simulink model "viewer_simulink"  (R2023a)
settings: Solver=VariableStepAuto  StartTime=0.0  StopTime=inf  RelTol=1e-3
undefined symbols (not defined in the file or in its folder): hl2ss
libraries: matrix_library x14, visionsinks x9, visionanalysis x4
settings Model: Creator=jcds  LastModifiedBy=jcds

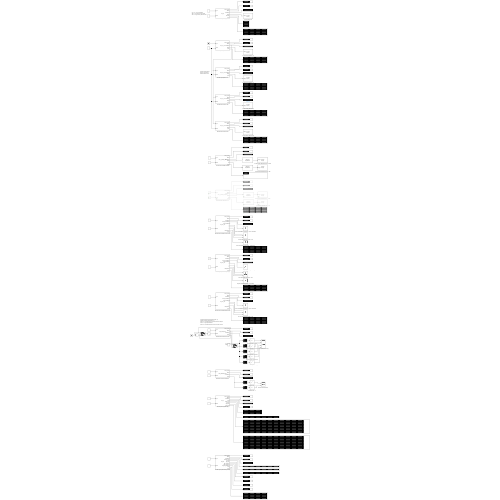
[thumbnail: Simulink's stored preview of the top-level diagram]
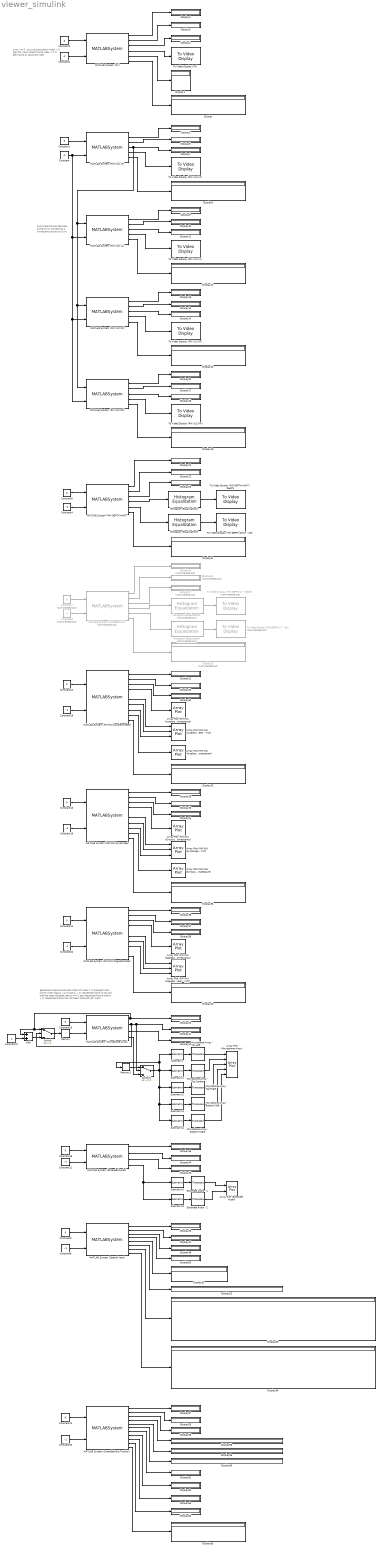
== system viewer_simulink ==
  note: Sequential capture example (start at index = 0)
      | Request next frame when status <= 0
      | status < 0: requested frame is too old and has been dropped
      | status == 0: got requested frame
      | status < 0: requested frame has not been received yet (wait)
  note: Associate frames between streams by connecting a timestamp output to sync
  note: sync <= 0 : no synchronization
      | index < 0: get nth most recent frame
      | index >= 0: get frame by absolute index
  Add : Sum
  Array Plot (Extended Audio) : ArrayPlot  NumInputPorts=2  WindowPosition=[158.000000,113.000000,800.000000,500.000000,]  Visible=on  ScopeFrameLocation=window  YLimits=[-0.0094,0.0077]  ShowLegend=on
  Array Plot (Microphone Array) : ArrayPlot  NumInputPorts=5  WindowPosition=[1013.000000,246.000000,800.000000,500.000000,]  Visible=on  ScopeFrameLocation=window  YLimits=[-0.0014,0.002]  ShowLegend=on
  Array Plot (RM IMU Accelerometer - Temperature) : ArrayPlot  WindowPosition=[770.000000,171.000000,800.000000,456.000000,]  Visible=on  ScopeFrameLocation=window  YLimits=[42.1563,54.2813]
  Array Plot (RM IMU Accelerometer - XYZ) : ArrayPlot  NumInputPorts=3  WindowPosition=[710.000000,401.000000,800.000000,500.000000,]  Visible=on  ScopeFrameLocation=window  YLimits=[-2.1398,11.1348]  ShowLegend=on
  Array Plot (RM IMU Accelerometer - sensor_timestamp) : ArrayPlot  WindowPosition=[1090.000000,48.000000,800.000000,456.000000,]  Visible=on  ScopeFrameLocation=window  YLimits=[302887973136.125,302992202644.875]
  Array Plot (RM IMU Gyroscope - Temperature) : ArrayPlot  WindowPosition=[770.000000,171.000000,800.000000,456.000000,]  Visible=on  ScopeFrameLocation=window  YLimits=[37.4858,48.2212]
  Array Plot (RM IMU Gyroscope - XYZ) : ArrayPlot  NumInputPorts=3  WindowPosition=[692.000000,115.000000,800.000000,500.000000,]  Visible=on  ScopeFrameLocation=window  YLimits=[-0.1057,0.1007]  ShowLegend=on
  Array Plot (RM IMU Gyroscope - sensor_timestamp) : ArrayPlot  WindowPosition=[1090.000000,48.000000,800.000000,456.000000,]  Visible=on  ScopeFrameLocation=window  YLimits=[302821386482.875,302881349464.125]
  Array Plot (RM IMU Magnetometer - XYZ) : ArrayPlot  NumInputPorts=3  WindowPosition=[952.000000,106.000000,800.000000,500.000000,]  Visible=on  ScopeFrameLocation=window  YLimits=[-377.475,569.775]  ShowLegend=on
  Array Plot (RM IMU Magnetometer - sensor_timestamp) : ArrayPlot  WindowPosition=[983.000000,49.000000,800.000000,456.000000,]  Visible=on  ScopeFrameLocation=window  YLimits=[302697878061.125,302947875559.875]
  Constant{,2,4,8,10,18..21} (9 alike) : Constant  Value=-1
  Constant{1,3,5,9,11..16} (10 alike) : Constant  Value=0
  Constant17 : Constant  OutDataTypeStr=int64
  Constant6 : Constant  Commented=on  Value=-1
  Constant7 : Constant  Commented=on  Value=0
  Display{,1..24,29..65} (62 alike) : Display
  Display{25..28} (4 alike) : Display  Commented=on
  Extended Audio - 1 : matrix_library/Transpose
  Extended Audio - 2 : matrix_library/Transpose
  Histogram Equalization : visionanalysis/Histogram Equalization  Commented=on  specify=Uniform  numbins=64  src=Specify via dialog  hist=ones(1,64)
  Histogram Equalization1 : visionanalysis/Histogram Equalization  Commented=on  specify=Uniform  numbins=64  src=Specify via dialog  hist=ones(1,64)
  Histogram Equalization2 : visionanalysis/Histogram Equalization  specify=Uniform  numbins=64  src=Specify via dialog  hist=ones(1,64)
  Histogram Equalization3 : visionanalysis/Histogram Equalization  specify=Uniform  numbins=64  src=Specify via dialog  hist=ones(1,64)
  MATLAB System (Extended Audio) : MATLABSystem  System=hl2ss.ms.sink_extended_audio  host=192.168.1.7  port=hl2ss.stream_port.EXTENDED_AUDIO  chunk=4096  mixer_mode=hl2ss.mixer_mode.BOTH  device=-1  loopback_gain=1.0  microphone_gain=1.0  profile=hl2ss.audio_profile.AAC_24000  level=hl2ss.aac_level.L2  buffer_size=1000  sample_time=hl2ss.parameters_microphone.GROUP_SIZE_AAC / hl2ss.parameters_microphone.SAMPLE_RATE  time_preference=hl2ss.grab_preference.PREFER_NEAREST  tiebreak_right=false  SimulateUsing=Code generation
      mask Type: hl2ss.ms.sink_extended_audio
      mask Display:
      | disp('sink_extended_audio');
      | port_label('input',1,'sync');
      | port_label('input',2,'index');
      | port_label('output',1,'frame_index');
      | port_label('output',2,'status');
      | port_label('output',3,'timestamp');
      | port_label('output',4,'audio');
  MATLAB System (Extended Eye Tracker) : MATLABSystem  System=hl2ss.ms.sink_eet  host=192.168.1.7  port=hl2ss.stream_port.EXTENDED_EYE_TRACKER  chunk=4096  framerate=90  buffer_size=300  sample_time=1 / 90  time_preference=hl2ss.grab_preference.PREFER_NEAREST  tiebreak_right=false  SimulateUsing=Code generation
      mask Type: hl2ss.ms.sink_eet
      mask Display:
      | disp('sink_eet');
      | port_label('input',1,'sync');
      | port_label('input',2,'index');
      | port_label('output',1,'frame_index');
      | port_label('output',2,'status');
      | port_label('output',3,'timestamp');
      | port_label('output',4,'combined_ray');
      | port_label('output',5,'left_ray');
      | port_label('output',6,'right_ray');
      | port_label('output',7,'left_openness');
      | port_label('output',8,'right_openness');
      | port_label('output',9,'vergence_distance');
      | port_label('output',10,'valid');
      | port_label('output',11,'pose');
  MATLAB System (Microphone Array) : MATLABSystem  System=hl2ss.ms.sink_microphone  host=192.168.1.7  port=hl2ss.stream_port.MICROPHONE  chunk=4096  profile=hl2ss.audio_profile.RAW  level=hl2ss.aac_level.L5  buffer_size=1000  sample_time=hl2ss.parameters_microphone.GROUP_SIZE_RAW / hl2ss.parameters_microphone.SAMPLE_RATE  time_preference=hl2ss.grab_preference.PREFER_NEAREST  tiebreak_right=false  SimulateUsing=Code generation
      mask Type: hl2ss.ms.sink_microphone
      mask Display:
      | disp('sink_microphone');
      | port_label('input',1,'sync');
      | port_label('input',2,'index');
      | port_label('output',1,'frame_index');
      | port_label('output',2,'status');
      | port_label('output',3,'timestamp');
      | port_label('output',4,'audio');
  MATLAB System (PV) : MATLABSystem  System=hl2ss.ms.sink_pv  host=192.168.1.7  port=hl2ss.stream_port.PERSONAL_VIDEO  width=640  height=360  framerate=30  chunk=4096  mode=hl2ss.stream_mode.MODE_1  divisor=1  profile=hl2ss.video_profile.H265_MAIN  level=hl2ss.h26x_level.DEFAULT  bitrate=0  options=[ hl2ss.h26x_encoder_property.CODECAPI_AVEncMPVGOPSize, 30 ]  decoded_format=hl2ss.pv_decoded_format.RGB  buffer_size=30 * 10  sample_time=1 / 30  enable_mrc=false  hologram_composition=true  recording_indicator=false  video_stabilization=false  blank_protected=false  show_mesh=false  shared=false  global_opacity=0.9  output_width=0.0  output_height=0.0  video_stabilization_length=0  hologram_perspective=hl2ss.hologram_perspective.PV  time_preference=hl2ss.grab_preference.PREFER_NEAREST  tiebreak_right=false  SimulateUsing=Code generation
      mask Type: hl2ss.ms.sink_pv
      mask Display:
      | disp('sink_pv');
      | port_label('input',1,'sync');
      | port_label('input',2,'index');
      | port_label('output',1,'frame_index');
      | port_label('output',2,'status');
      | port_label('output',3,'timestamp');
      | port_label('output',4,'image');
      | port_label('output',5,'intrinsics');
      | port_label('output',6,'pose');
  MATLAB System (RM DEPTH AHAT) : MATLABSystem  System=hl2ss.ms.sink_rm_depth_ahat  host=192.168.1.7  port=hl2ss.stream_port.RM_DEPTH_AHAT  chunk=4096  mode=hl2ss.stream_mode.MODE_1  divisor=1  profile_z=hl2ss.depth_profile.SAME  profile_ab=hl2ss.video_profile.H265_MAIN  level=hl2ss.h26x_level.DEFAULT  bitrate=0  options=[ hl2ss.h26x_encoder_property.CODECAPI_AVEncMPVGOPSize, hl2ss.parameters_rm_depth_ahat.FPS ]  buffer_size=hl2ss.parameters_rm_depth_ahat.FPS * 10  sample_time=1 / hl2ss.parameters_rm_depth_ahat.FPS  time_preference=hl2ss.grab_preference.PREFER_NEAREST  tiebreak_right=false  SimulateUsing=Code generation
      mask Type: hl2ss.ms.sink_rm_depth_ahat
      mask Display:
      | disp('sink_rm_depth_ahat');
      | port_label('input',1,'sync');
      | port_label('input',2,'index');
      | port_label('output',1,'frame_index');
      | port_label('output',2,'status');
      | port_label('output',3,'timestamp');
      | port_label('output',4,'depth');
      | port_label('output',5,'ab');
      | port_label('output',6,'pose');
  MATLAB System (RM DEPTH LT) : MATLABSystem  Commented=on  System=hl2ss.ms.sink_rm_depth_longthrow  host=192.168.1.7  port=hl2ss.stream_port.RM_DEPTH_LONGTHROW  chunk=4096  mode=hl2ss.stream_mode.MODE_1  divisor=1  png_filter=hl2ss.png_filter_mode.PAETH  buffer_size=hl2ss.parameters_rm_depth_longthrow.FPS * 10  sample_time=1 / hl2ss.parameters_rm_depth_longthrow.FPS  time_preference=hl2ss.grab_preference.PREFER_NEAREST  tiebreak_right=false  SimulateUsing=Code generation
      mask Type: hl2ss.ms.sink_rm_depth_longthrow
      mask Display:
      | disp('sink_rm_depth_longthrow');
      | port_label('input',1,'sync');
      | port_label('input',2,'index');
      | port_label('output',1,'frame_index');
      | port_label('output',2,'status');
      | port_label('output',3,'timestamp');
      | port_label('output',4,'depth');
      | port_label('output',5,'ab');
      | port_label('output',6,'pose');
  MATLAB System (RM IMU Accelerometer) : MATLABSystem  System=hl2ss.ms.sink_rm_imu  host=192.168.1.7  port=hl2ss.stream_port.RM_IMU_ACCELEROMETER  chunk=4096  mode=hl2ss.stream_mode.MODE_1  buffer_size=300  sample_time=1 / 30  time_preference=hl2ss.grab_preference.PREFER_NEAREST  tiebreak_right=false  SimulateUsing=Code generation
      mask Type: hl2ss.ms.sink_rm_imu
      mask Display:
      | disp('sink_rm_imu');
      | port_label('input',1,'sync');
      | port_label('input',2,'index');
      | port_label('output',1,'frame_index');
      | port_label('output',2,'status');
      | port_label('output',3,'timestamp');
      | port_label('output',4,'sensor_timestamp');
      | port_label('output',5,'host_timestamp');
      | port_label('output',6,'x');
      | port_label('output',7,'y');
      | port_label('output',8,'z');
      | port_label('output',9,'temperature');
      | port_label('output',10,'pose');
  MATLAB System (RM IMU Gyroscope) : MATLABSystem  System=hl2ss.ms.sink_rm_imu  host=192.168.1.7  port=hl2ss.stream_port.RM_IMU_GYROSCOPE  chunk=4096  mode=hl2ss.stream_mode.MODE_1  buffer_size=300  sample_time=1 / 30  time_preference=hl2ss.grab_preference.PREFER_NEAREST  tiebreak_right=false  SimulateUsing=Code generation
      mask Type: hl2ss.ms.sink_rm_imu
      mask Display:
      | disp('sink_rm_imu');
      | port_label('input',1,'sync');
      | port_label('input',2,'index');
      | port_label('output',1,'frame_index');
      | port_label('output',2,'status');
      | port_label('output',3,'timestamp');
      | port_label('output',4,'sensor_timestamp');
      | port_label('output',5,'host_timestamp');
      | port_label('output',6,'x');
      | port_label('output',7,'y');
      | port_label('output',8,'z');
      | port_label('output',9,'temperature');
      | port_label('output',10,'pose');
  MATLAB System (RM IMU Magnetometer) : MATLABSystem  System=hl2ss.ms.sink_rm_imu  host=192.168.1.7  port=hl2ss.stream_port.RM_IMU_MAGNETOMETER  chunk=4096  mode=hl2ss.stream_mode.MODE_1  buffer_size=300  sample_time=1 / 30  time_preference=hl2ss.grab_preference.PREFER_NEAREST  tiebreak_right=false  SimulateUsing=Code generation
      mask Type: hl2ss.ms.sink_rm_imu
      mask Display:
      | disp('sink_rm_imu');
      | port_label('input',1,'sync');
      | port_label('input',2,'index');
      | port_label('output',1,'frame_index');
      | port_label('output',2,'status');
      | port_label('output',3,'timestamp');
      | port_label('output',4,'sensor_timestamp');
      | port_label('output',5,'host_timestamp');
      | port_label('output',6,'x');
      | port_label('output',7,'y');
      | port_label('output',8,'z');
      | port_label('output',9,'temperature');
      | port_label('output',10,'pose');
  MATLAB System (RM VLC LF) : MATLABSystem  System=hl2ss.ms.sink_rm_vlc  host=192.168.1.7  port=hl2ss.stream_port.RM_VLC_LEFTFRONT  chunk=4096  mode=hl2ss.stream_mode.MODE_1  divisor=1  profile=hl2ss.video_profile.H265_MAIN  level=hl2ss.h26x_level.DEFAULT  bitrate=0  options=[ hl2ss.h26x_encoder_property.CODECAPI_AVEncMPVGOPSize, 30 ]  buffer_size=300  sample_time=1 / 30  time_preference=hl2ss.grab_preference.PREFER_NEAREST  tiebreak_right=false  SimulateUsing=Code generation
      mask Type: hl2ss.ms.sink_rm_vlc
      mask Display:
      | disp('sink_rm_vlc');
      | port_label('input',1,'sync');
      | port_label('input',2,'index');
      | port_label('output',1,'frame_index');
      | port_label('output',2,'status');
      | port_label('output',3,'timestamp');
      | port_label('output',4,'image');
      | port_label('output',5,'pose');
  MATLAB System (RM VLC LL) : MATLABSystem  System=hl2ss.ms.sink_rm_vlc  host=192.168.1.7  port=hl2ss.stream_port.RM_VLC_LEFTLEFT  chunk=4096  mode=hl2ss.stream_mode.MODE_1  divisor=1  profile=hl2ss.video_profile.H265_MAIN  level=hl2ss.h26x_level.DEFAULT  bitrate=0  options=[ hl2ss.h26x_encoder_property.CODECAPI_AVEncMPVGOPSize, 30 ]  buffer_size=300  sample_time=1 / 30  time_preference=hl2ss.grab_preference.PREFER_NEAREST  tiebreak_right=false  SimulateUsing=Code generation
      mask Type: hl2ss.ms.sink_rm_vlc
      mask Display:
      | disp('sink_rm_vlc');
      | port_label('input',1,'sync');
      | port_label('input',2,'index');
      | port_label('output',1,'frame_index');
      | port_label('output',2,'status');
      | port_label('output',3,'timestamp');
      | port_label('output',4,'image');
      | port_label('output',5,'pose');
  MATLAB System (RM VLC RF) : MATLABSystem  System=hl2ss.ms.sink_rm_vlc  host=192.168.1.7  port=hl2ss.stream_port.RM_VLC_RIGHTFRONT  chunk=4096  mode=hl2ss.stream_mode.MODE_1  divisor=1  profile=hl2ss.video_profile.H265_MAIN  level=hl2ss.h26x_level.DEFAULT  bitrate=0  options=[ hl2ss.h26x_encoder_property.CODECAPI_AVEncMPVGOPSize, 30 ]  buffer_size=300  sample_time=1 / 30  time_preference=hl2ss.grab_preference.PREFER_NEAREST  tiebreak_right=false  SimulateUsing=Code generation
      mask Type: hl2ss.ms.sink_rm_vlc
      mask Display:
      | disp('sink_rm_vlc');
      | port_label('input',1,'sync');
      | port_label('input',2,'index');
      | port_label('output',1,'frame_index');
      | port_label('output',2,'status');
      | port_label('output',3,'timestamp');
      | port_label('output',4,'image');
      | port_label('output',5,'pose');
  MATLAB System (RM VLC RR) : MATLABSystem  System=hl2ss.ms.sink_rm_vlc  host=192.168.1.7  port=hl2ss.stream_port.RM_VLC_RIGHTRIGHT  chunk=4096  mode=hl2ss.stream_mode.MODE_1  divisor=1  profile=hl2ss.video_profile.H265_MAIN  level=hl2ss.h26x_level.DEFAULT  bitrate=0  options=[ hl2ss.h26x_encoder_property.CODECAPI_AVEncMPVGOPSize, 30 ]  buffer_size=300  sample_time=1 / 30  time_preference=hl2ss.grab_preference.PREFER_NEAREST  tiebreak_right=false  SimulateUsing=Code generation
      mask Type: hl2ss.ms.sink_rm_vlc
      mask Display:
      | disp('sink_rm_vlc');
      | port_label('input',1,'sync');
      | port_label('input',2,'index');
      | port_label('output',1,'frame_index');
      | port_label('output',2,'status');
      | port_label('output',3,'timestamp');
      | port_label('output',4,'image');
      | port_label('output',5,'pose');
  MATLAB System (Spatial Input) : MATLABSystem  System=hl2ss.ms.sink_si  host=192.168.1.7  port=hl2ss.stream_port.SPATIAL_INPUT  chunk=4096  buffer_size=300  sample_time=1 / hl2ss.parameters_si.SAMPLE_RATE  time_preference=hl2ss.grab_preference.PREFER_NEAREST  tiebreak_right=false  SimulateUsing=Code generation
      mask Type: hl2ss.ms.sink_si
      mask Display:
      | disp('sink_si');
      | port_label('input',1,'sync');
      | port_label('input',2,'index');
      | port_label('output',1,'frame_index');
      | port_label('output',2,'status');
      | port_label('output',3,'timestamp');
      | port_label('output',4,'valid');
      | port_label('output',5,'head_pose');
      | port_label('output',6,'eye_ray');
      | port_label('output',7,'left_hand');
      | port_label('output',8,'right_hand');
  Memory : Memory
  Memory1 : Memory
  Microphone Array - Bottom Left : matrix_library/Transpose
  Microphone Array - Bottom Right : matrix_library/Transpose
  Microphone Array - Top Center : matrix_library/Transpose
  Microphone Array - Top Left : matrix_library/Transpose
  Microphone Array - Top Right : matrix_library/Transpose
  Submatrix : matrix_library/Submatrix  RowSpan=One row  RowStartMode=Index  RowStartIndex=1  RowEndMode=Last  RowEndIndex=1  ColSpan=All columns  ColStartMode=First  ColStartIndex=1  ColEndMode=Last  ColEndIndex=1
  Submatrix1 : matrix_library/Submatrix  RowSpan=One row  RowStartMode=Index  RowStartIndex=2  RowEndMode=Last  RowEndIndex=1  ColSpan=All columns  ColStartMode=First  ColStartIndex=1  ColEndMode=Last  ColEndIndex=1
  Submatrix2 : matrix_library/Submatrix  RowSpan=One row  RowStartMode=Index  RowStartIndex=3  RowEndMode=Last  RowEndIndex=1  ColSpan=All columns  ColStartMode=First  ColStartIndex=1  ColEndMode=Last  ColEndIndex=1
  Submatrix3 : matrix_library/Submatrix  RowSpan=One row  RowStartMode=Index  RowStartIndex=4  RowEndMode=Last  RowEndIndex=1  ColSpan=All columns  ColStartMode=First  ColStartIndex=1  ColEndMode=Last  ColEndIndex=1
  Submatrix4 : matrix_library/Submatrix  RowSpan=One row  RowStartMode=Index  RowStartIndex=5  RowEndMode=Last  RowEndIndex=1  ColSpan=All columns  ColStartMode=First  ColStartIndex=1  ColEndMode=Last  ColEndIndex=1
  Submatrix5 : matrix_library/Submatrix  RowSpan=One row  RowStartMode=Index  RowStartIndex=1  RowEndMode=Last  RowEndIndex=1  ColSpan=All columns  ColStartMode=First  ColStartIndex=1  ColEndMode=Last  ColEndIndex=1
  Submatrix6 : matrix_library/Submatrix  RowSpan=One row  RowStartMode=Index  RowStartIndex=2  RowEndMode=Last  RowEndIndex=1  ColSpan=All columns  ColStartMode=First  ColStartIndex=1  ColEndMode=Last  ColEndIndex=1
  Switch : Switch  Criteria=u2 > Threshold  SaturateOnIntegerOverflow=off  InputSameDT=off
  Switch1 : Switch  Criteria=u2 ~= 0  SaturateOnIntegerOverflow=off  InputSameDT=off
  To Video Display (PV) : visionsinks/To Video Display  windowSizeMode=Normal  openAtMdlStart=on  fullScreen=off  videoWindowX=2170  videoWindowY=212  saveWindowSize=off  videoWindowWidth=640  videoWindowHeight=360  inputColorFormat=RGB  inputType=Obsolete  imagePorts=One multidimensional signal  OutputDevice=On-screen video monitor  dataOrg=Column-major  isWindowOpen=off
  To Video Display (RM DEPTH AHAT - AB) : visionsinks/To Video Display  windowSizeMode=Normal  openAtMdlStart=on  fullScreen=off  videoWindowX=2573  videoWindowY=991  saveWindowSize=off  videoWindowWidth=744  videoWindowHeight=668  inputColorFormat=RGB  inputType=Obsolete  imagePorts=One multidimensional signal  OutputDevice=On-screen video monitor  dataOrg=Column-major  isWindowOpen=off
  To Video Display (RM DEPTH AHAT - Depth) : visionsinks/To Video Display  windowSizeMode=Normal  openAtMdlStart=on  fullScreen=off  videoWindowX=1597  videoWindowY=1025  saveWindowSize=off  videoWindowWidth=829  videoWindowHeight=727  inputColorFormat=RGB  inputType=Obsolete  imagePorts=One multidimensional signal  OutputDevice=On-screen video monitor  dataOrg=Column-major  isWindowOpen=off
  To Video Display (RM DEPTH LT - AB) : visionsinks/To Video Display  Commented=on  windowSizeMode=Normal  openAtMdlStart=on  fullScreen=off  videoWindowX=917  videoWindowY=1195  saveWindowSize=off  videoWindowWidth=512  videoWindowHeight=512  inputColorFormat=RGB  inputType=Obsolete  imagePorts=One multidimensional signal  OutputDevice=On-screen video monitor  dataOrg=Column-major  isWindowOpen=off
  To Video Display (RM DEPTH LT - Depth) : visionsinks/To Video Display  Commented=on  windowSizeMode=Normal  openAtMdlStart=on  fullScreen=off  videoWindowX=1462  videoWindowY=1164  saveWindowSize=off  videoWindowWidth=512  videoWindowHeight=512  inputColorFormat=RGB  inputType=Obsolete  imagePorts=One multidimensional signal  OutputDevice=On-screen video monitor  dataOrg=Column-major  isWindowOpen=off
  To Video Display (RM VLC LF) : visionsinks/To Video Display  windowSizeMode=Normal  openAtMdlStart=on  fullScreen=off  videoWindowX=2960  videoWindowY=641  saveWindowSize=off  videoWindowWidth=781  videoWindowHeight=480  inputColorFormat=RGB  inputType=Obsolete  imagePorts=One multidimensional signal  OutputDevice=On-screen video monitor  dataOrg=Column-major  isWindowOpen=off
  To Video Display (RM VLC LL) : visionsinks/To Video Display  windowSizeMode=Normal  openAtMdlStart=on  fullScreen=off  videoWindowX=2971  videoWindowY=101  saveWindowSize=off  videoWindowWidth=781  videoWindowHeight=480  inputColorFormat=RGB  inputType=Obsolete  imagePorts=One multidimensional signal  OutputDevice=On-screen video monitor  dataOrg=Column-major  isWindowOpen=off
  To Video Display (RM VLC RF) : visionsinks/To Video Display  windowSizeMode=Normal  openAtMdlStart=on  fullScreen=off  videoWindowX=2330  videoWindowY=1248  saveWindowSize=off  videoWindowWidth=781  videoWindowHeight=480  inputColorFormat=RGB  inputType=Obsolete  imagePorts=One multidimensional signal  OutputDevice=On-screen video monitor  dataOrg=Column-major  isWindowOpen=off
  To Video Display (RM VLC RR) : visionsinks/To Video Display  windowSizeMode=Normal  openAtMdlStart=on  fullScreen=off  videoWindowX=2962  videoWindowY=1176  saveWindowSize=off  videoWindowWidth=781  videoWindowHeight=480  inputColorFormat=RGB  inputType=Obsolete  imagePorts=One multidimensional signal  OutputDevice=On-screen video monitor  dataOrg=Column-major  isWindowOpen=off
  wires:
  MATLAB System (PV)/4 -> To Video Display (PV)/1
  MATLAB System (PV)/6 -> Display/1
  MATLAB System (PV)/5 -> Display1/1
  MATLAB System (PV)/3 -> Display2/1
  MATLAB System (PV)/2 -> Display3/1
  MATLAB System (PV)/1 -> Display4/1
  MATLAB System (RM VLC LF)/4 -> To Video Display (RM VLC LF)/1
  MATLAB System (RM VLC LF)/1 -> Display5/1
  MATLAB System (RM VLC LF)/2 -> Display6/1
  MATLAB System (RM VLC LF)/3 -> MATLAB System (RM VLC RR)/1, MATLAB System (RM VLC RF)/1, MATLAB System (RM VLC LL)/1, Display7/1
  MATLAB System (RM VLC LF)/5 -> Display8/1
  MATLAB System (RM VLC LL)/5 -> Display12/1
  MATLAB System (RM VLC LL)/3 -> Display11/1
  MATLAB System (RM VLC LL)/4 -> To Video Display (RM VLC LL)/1
  MATLAB System (RM VLC LL)/2 -> Display10/1
  MATLAB System (RM VLC LL)/1 -> Display9/1
  MATLAB System (RM VLC RF)/3 -> Display14/1
  MATLAB System (RM VLC RF)/4 -> To Video Display (RM VLC RF)/1
  MATLAB System (RM VLC RF)/1 -> Display16/1
  MATLAB System (RM VLC RF)/2 -> Display13/1
  MATLAB System (RM VLC RF)/5 -> Display15/1
  MATLAB System (RM VLC RR)/3 -> Display18/1
  MATLAB System (RM VLC RR)/1 -> Display20/1
  MATLAB System (RM VLC RR)/4 -> To Video Display (RM VLC RR)/1
  MATLAB System (RM VLC RR)/5 -> Display19/1
  MATLAB System (RM VLC RR)/2 -> Display17/1
  MATLAB System (RM DEPTH AHAT)/6 -> Display21/1
  MATLAB System (RM DEPTH AHAT)/2 -> Display22/1
  MATLAB System (RM DEPTH AHAT)/3 -> Display23/1
  MATLAB System (RM DEPTH AHAT)/1 -> Display24/1
  MATLAB System (RM DEPTH LT)/2 -> Display26/1
  MATLAB System (RM DEPTH LT)/1 -> Display28/1
  MATLAB System (RM DEPTH LT)/6 -> Display25/1
  MATLAB System (RM DEPTH LT)/3 -> Display27/1
  MATLAB System (RM DEPTH LT)/5 -> Histogram Equalization/1
  Histogram Equalization/1 -> To Video Display (RM DEPTH LT - AB)/1
  Histogram Equalization1/1 -> To Video Display (RM DEPTH LT - Depth)/1
  MATLAB System (RM DEPTH LT)/4 -> Histogram Equalization1/1
  Histogram Equalization2/1 -> To Video Display (RM DEPTH AHAT - Depth)/1
  Histogram Equalization3/1 -> To Video Display (RM DEPTH AHAT - AB)/1
  MATLAB System (RM DEPTH AHAT)/4 -> Histogram Equalization2/1
  MATLAB System (RM DEPTH AHAT)/5 -> Histogram Equalization3/1
  MATLAB System (RM IMU Accelerometer)/1 -> Display31/1
  MATLAB System (RM IMU Accelerometer)/2 -> Display29/1
  MATLAB System (RM IMU Accelerometer)/3 -> Display30/1
  MATLAB System (RM IMU Accelerometer)/6 -> Array Plot (RM IMU Accelerometer - XYZ)/1
  MATLAB System (RM IMU Accelerometer)/7 -> Array Plot (RM IMU Accelerometer - XYZ)/2
  MATLAB System (RM IMU Accelerometer)/8 -> Array Plot (RM IMU Accelerometer - XYZ)/3
  MATLAB System (RM IMU Accelerometer)/9 -> Array Plot (RM IMU Accelerometer - Temperature)/1
  MATLAB System (RM IMU Accelerometer)/10 -> Display32/1
  MATLAB System (RM IMU Accelerometer)/4 -> Array Plot (RM IMU Accelerometer - sensor_timestamp)/1
  MATLAB System (RM IMU Gyroscope)/6 -> Array Plot (RM IMU Gyroscope - XYZ)/1
  MATLAB System (RM IMU Gyroscope)/1 -> Display35/1
  MATLAB System (RM IMU Gyroscope)/7 -> Array Plot (RM IMU Gyroscope - XYZ)/2
  MATLAB System (RM IMU Gyroscope)/8 -> Array Plot (RM IMU Gyroscope - XYZ)/3
  MATLAB System (RM IMU Gyroscope)/4 -> Array Plot (RM IMU Gyroscope - sensor_timestamp)/1
  MATLAB System (RM IMU Gyroscope)/10 -> Display36/1
  MATLAB System (RM IMU Gyroscope)/9 -> Array Plot (RM IMU Gyroscope - Temperature)/1
  MATLAB System (RM IMU Gyroscope)/3 -> Display34/1
  MATLAB System (RM IMU Gyroscope)/2 -> Display33/1
  MATLAB System (RM IMU Magnetometer)/4 -> Array Plot (RM IMU Magnetometer - sensor_timestamp)/1
  MATLAB System (RM IMU Magnetometer)/2 -> Display37/1
  MATLAB System (RM IMU Magnetometer)/3 -> Display38/1
  MATLAB System (RM IMU Magnetometer)/1 -> Display39/1
  MATLAB System (RM IMU Magnetometer)/8 -> Array Plot (RM IMU Magnetometer - XYZ)/3
  MATLAB System (RM IMU Magnetometer)/10 -> Display40/1
  MATLAB System (RM IMU Magnetometer)/6 -> Array Plot (RM IMU Magnetometer - XYZ)/1
  MATLAB System (RM IMU Magnetometer)/7 -> Array Plot (RM IMU Magnetometer - XYZ)/2
  MATLAB System (Microphone Array)/1 -> Add/1, Switch/1, Display43/1
  MATLAB System (Microphone Array)/3 -> Display42/1
  Submatrix/1 -> Microphone Array - Top Left/1
  Microphone Array - Top Left/1 -> Array Plot (Microphone Array)/1
  Submatrix1/1 -> Microphone Array - Top Center/1
  Submatrix2/1 -> Microphone Array - Top Right/1
  Submatrix3/1 -> Microphone Array - Bottom Left/1
  Submatrix4/1 -> Microphone Array - Bottom Right/1
  Microphone Array - Top Center/1 -> Array Plot (Microphone Array)/2
  Microphone Array - Top Right/1 -> Array Plot (Microphone Array)/3
  Microphone Array - Bottom Left/1 -> Array Plot (Microphone Array)/4
  Microphone Array - Bottom Right/1 -> Array Plot (Microphone Array)/5
  MATLAB System (Extended Audio)/1 -> Display46/1
  Submatrix6/1 -> Extended Audio - 2/1
  Submatrix5/1 -> Extended Audio - 1/1
  MATLAB System (Extended Audio)/2 -> Display44/1
  MATLAB System (Extended Audio)/3 -> Display45/1
  Extended Audio - 1/1 -> Array Plot (Extended Audio)/1
  Extended Audio - 2/1 -> Array Plot (Extended Audio)/2
  MATLAB System (Extended Audio)/4 -> Submatrix6/1, Submatrix5/1
  MATLAB System (Spatial Input)/1 -> Display49/1
  MATLAB System (Spatial Input)/2 -> Display47/1
  MATLAB System (Spatial Input)/3 -> Display48/1
  MATLAB System (Spatial Input)/4 -> Display50/1
  MATLAB System (Spatial Input)/5 -> Display51/1
  MATLAB System (Spatial Input)/6 -> Display52/1
  MATLAB System (Spatial Input)/7 -> Display53/1
  MATLAB System (Spatial Input)/8 -> Display54/1
  MATLAB System (Extended Eye Tracker)/1 -> Display57/1
  MATLAB System (Extended Eye Tracker)/2 -> Display55/1
  MATLAB System (Extended Eye Tracker)/3 -> Display56/1
  MATLAB System (Extended Eye Tracker)/4 -> Display58/1
  MATLAB System (Extended Eye Tracker)/5 -> Display59/1
  MATLAB System (Extended Eye Tracker)/6 -> Display60/1
  MATLAB System (Extended Eye Tracker)/7 -> Display61/1
  MATLAB System (Extended Eye Tracker)/8 -> Display62/1
  MATLAB System (Extended Eye Tracker)/9 -> Display63/1
  MATLAB System (Extended Eye Tracker)/10 -> Display64/1
  MATLAB System (Extended Eye Tracker)/11 -> Display65/1
  Constant/1 -> MATLAB System (RM VLC RR)/2, MATLAB System (RM VLC RF)/2, MATLAB System (RM VLC LL)/2, MATLAB System (RM VLC LF)/2
  Constant1/1 -> MATLAB System (RM VLC LF)/1
  Constant3/1 -> MATLAB System (PV)/1
  Constant2/1 -> MATLAB System (PV)/2
  Constant4/1 -> MATLAB System (RM DEPTH AHAT)/2
  Constant5/1 -> MATLAB System (RM DEPTH AHAT)/1
  Constant6/1 -> MATLAB System (RM DEPTH LT)/2
  Constant7/1 -> MATLAB System (RM DEPTH LT)/1
  Constant9/1 -> MATLAB System (Spatial Input)/1
  Constant8/1 -> MATLAB System (Spatial Input)/2
  Constant11/1 -> MATLAB System (Extended Eye Tracker)/1
  Constant10/1 -> MATLAB System (Extended Eye Tracker)/2
  Constant12/1 -> MATLAB System (RM IMU Accelerometer)/1
  Constant13/1 -> MATLAB System (RM IMU Gyroscope)/1
  Constant14/1 -> MATLAB System (RM IMU Magnetometer)/1
  Constant15/1 -> MATLAB System (Microphone Array)/1
  Constant16/1 -> MATLAB System (Extended Audio)/1
  Constant17/1 -> Add/2
  Switch/1 -> Memory/1
  Constant18/1 -> MATLAB System (RM IMU Accelerometer)/2
  Constant19/1 -> MATLAB System (RM IMU Gyroscope)/2
  Constant20/1 -> MATLAB System (RM IMU Magnetometer)/2
  Constant21/1 -> MATLAB System (Extended Audio)/2
  Memory/1 -> MATLAB System (Microphone Array)/2
  MATLAB System (Microphone Array)/2 -> Switch/2, Switch1/2, Display41/1
  Add/1 -> Switch/3
  MATLAB System (Microphone Array)/4 -> Switch1/3
  Memory1/1 -> Switch1/1
  Switch1/1 -> Submatrix1/1, Submatrix/1, Memory1/1, Submatrix4/1, Submatrix3/1, Submatrix2/1
